simulink model "Calibration_acceleration_brake"  (R2020b)
settings: Solver=VariableStepAuto  StartTime=0.0  StopTime=10  RelTol=1e-3
libraries: Solver_SF x1
settings Model: Creator=wwcong  LastModifiedBy=85304
settings DataIOCC: ReturnWorkspaceOutputs=off
settings DebuggingCC: ArithmeticOperatorsInVariantConditions=warning
settings SFSimCC: SimUseLocalCustomCode=off  CustomCodeUndefinedFunction=UseInterfaceOnly
settings RTWCC: RTWUseLocalCustomCode=off

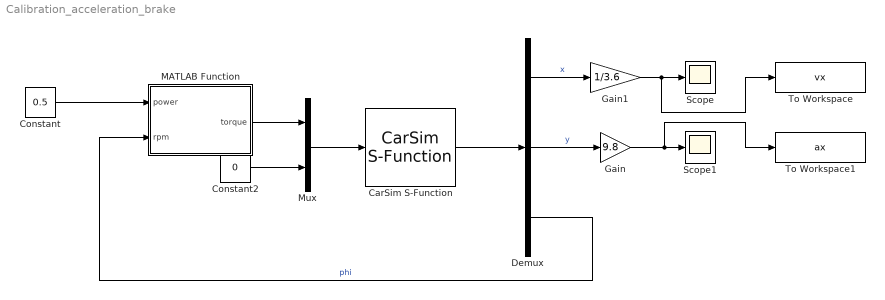
== system Calibration_acceleration_brake ==
  CarSim S-Function : Solver_SF/CarSim S-Function  Priority=1  SIMFILE=simfile.sim
  Constant : Constant  Value=0.5
  Constant2 : Constant  Value=0
  Demux : Demux  Outputs=3
  Gain : Gain  Gain=9.8
  Gain1 : Gain  Gain=1/3.6
  MATLAB Function : MATLAB Function  TreatAsAtomicUnit=on
  Mux : Mux  Inputs=2
  Scope : Scope
  Scope1 : Scope
  To Workspace : ToWorkspace  VariableName=vx  SaveFormat=Timeseries  SampleTime=-1
  To Workspace1 : ToWorkspace  VariableName=ax  SaveFormat=Timeseries  SampleTime=-1
  wires:
  CarSim S-Function/1 -> Demux/1
  MATLAB Function/1(torque) -> Mux/1
  Mux/1 -> CarSim S-Function/1
  Demux/1 -> Gain1/1  "x"
  Demux/2 -> Gain/1  "y"
  Demux/3 -> MATLAB Function/2(rpm)  "phi"
  Constant/1 -> MATLAB Function/1(power)
  Gain1/1 -> To Workspace/1, Scope/1
  Gain/1 -> To Workspace1/1, Scope1/1
  Constant2/1 -> Mux/2

== matlab function Calibration_acceleration_brake/MATLAB Function ==
  data: power input; torque output; rpm input
function torque = fcn(power,rpm)
Tmax=400*power;
if(rpm<4532)
    torque=Tmax;
else 
    torque=Tmax*4523/rpm;
end
end
